simulink model "verif_of_eom"  (R2017a)
settings: Solver=VariableStepAuto  StartTime=0.0  StopTime=10.0  RelTol=1e-5
settings Model: Creator=bacula2  LastModifiedBy=jabyrns2

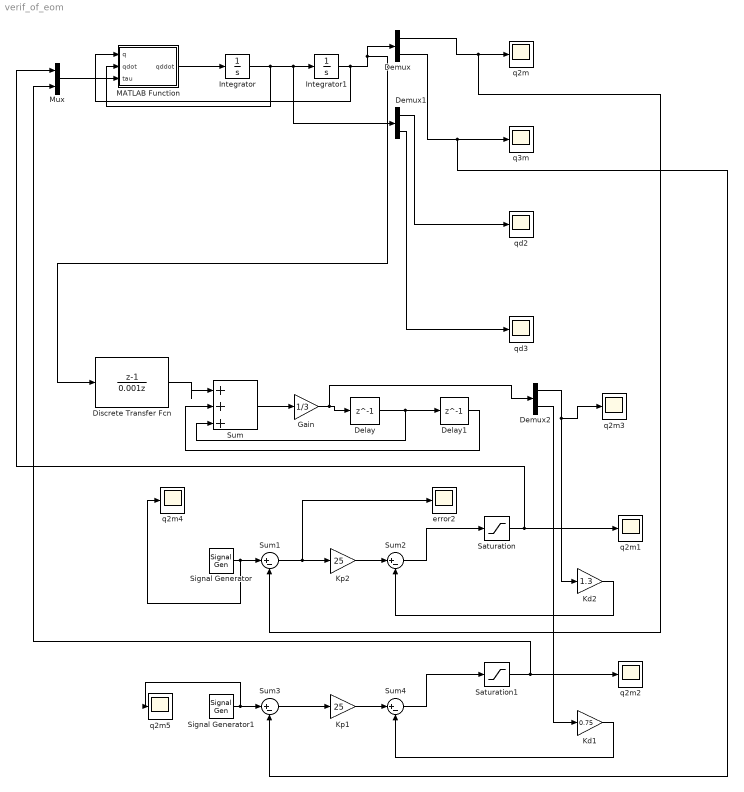
== system verif_of_eom ==
  Delay : Delay  DelayLength=1  InitialCondition=0  SampleTime=0.001
  Delay1 : Delay  DelayLength=1  InitialCondition=0  SampleTime=0.001
  Demux : Demux  Outputs=2
  Demux1 : Demux  Outputs=2
  Demux2 : Demux  Outputs=2
  Discrete Transfer Fcn : DiscreteTransferFcn  Numerator=[1 -1]  Denominator=[0.001 0]  SampleTime=0.001
  Gain : Gain  Gain=1/3
  Integrator : Integrator  InitialCondition=[0;0]
  Integrator1 : Integrator  InitialCondition=[0;0]
  Kd1 : Gain  Gain=0.75
  Kd2 : Gain  Gain=1.3
  Kp1 : Gain  Gain=25
  Kp2 : Gain  Gain=25
  MATLAB Function : MATLAB Function  TreatAsAtomicUnit=on
  Mux : Mux  Inputs=2
  Saturation : Saturate  UpperLimit=5  LowerLimit=-5
  Saturation1 : Saturate  UpperLimit=5  LowerLimit=-5
  Signal Generator : SignalGenerator  WaveForm=square  Amplitude=0.2  Frequency=0.5
  Signal Generator1 : SignalGenerator  WaveForm=square  Amplitude=0.2  Frequency=0.5
  Sum : Sum  Inputs=|+++
  Sum{1..4} (4 alike) : Sum  Inputs=|+-
  error2 : Scope
  q2m{,1..5} (6 alike) : Scope
  q3m : Scope
  qd2 : Scope
  qd3 : Scope
  wires:
  MATLAB Function/1(qddot) -> Integrator/1
  Integrator/1 -> MATLAB Function/2(qdot), Demux1/1, Integrator1/1
  Integrator1/1 -> MATLAB Function/1(q), Discrete Transfer Fcn/1, Demux/1
  Demux/1 -> Sum1/2, q2m/1
  Demux1/1 -> qd2/1
  Demux1/2 -> qd3/1
  Discrete Transfer Fcn/1 -> Sum/1
  Sum/1 -> Gain/1
  Gain/1 -> Demux2/1, Delay/1
  Delay/1 -> Sum/3, Delay1/1
  Delay1/1 -> Sum/2
  Signal Generator/1 -> q2m4/1, Sum1/1
  Demux2/1 -> q2m3/1, Kd2/1
  Sum1/1 -> error2/1, Kp2/1
  Kp2/1 -> Sum2/1
  Kd2/1 -> Sum2/2
  Sum2/1 -> Saturation/1
  Saturation/1 -> Mux/1, q2m1/1
  Sum4/1 -> Saturation1/1
  Saturation1/1 -> Mux/2, q2m2/1
  Demux2/2 -> Kd1/1
  Kp1/1 -> Sum4/1
  Demux/2 -> Sum3/2, q3m/1
  Sum3/1 -> Kp1/1
  Signal Generator1/1 -> q2m5/1, Sum3/1
  Kd1/1 -> Sum4/2
  Mux/1 -> MATLAB Function/3(tau)

== matlab function verif_of_eom/MATLAB Function ==
  data: q input; qddot output; qdot input; tau input
function qddot = fcn(q,qdot,tau)
q2 = q(1); q3 = q(2);
qd2 = qdot(1); qd3 = qdot(2);
p1 = 0.03;
p2 = 0.0128;
p3 = 0.0076;
p4 = 0.0753;
p5 = 0.0298;
g = 9.804;


D = [p1, -p3*sin(q3-q2); 
    -p3*sin(q3-q2), p2];

C = [0, -p3*cos(q3-q2)*qd3;
    p3*cos(q3-q2)*qd2, 0];

G = [-p4*g*sin(q2);
    -p5*g*cos(q3)];

qddot = D\(tau - G - C*qdot);
